simulink model "lyapunov_controller"  (R2016b)
settings: Solver=VariableStepAuto  StartTime=0.0  StopTime=200.0  RelTol=1e-3
libraries: simulink x2
settings Model: Creator=jocol  LastModifiedBy=jocol
settings DataIOCC: InspectSignalLogs=on

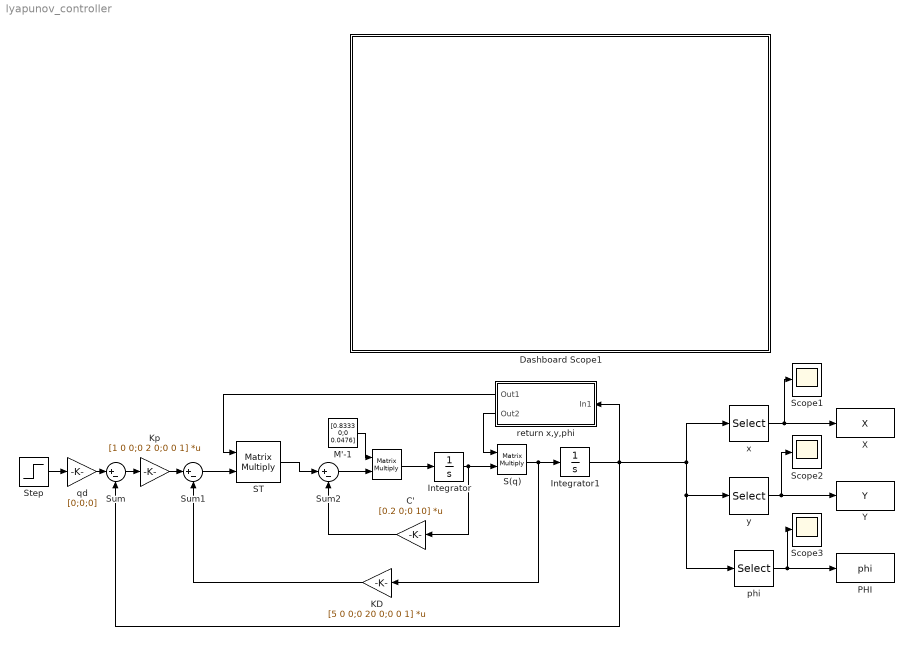
== system lyapunov_controller ==
  " " : Product  Multiplication=Matrix(*)
  C' : Gain  Gain=[0.2 0;0 10]  Multiplication=Matrix(K*u)
  Dashboard Scope1 : Subsystem  DialogController=hmiCreateDDGDialog  IsWebBlock=on  mask(MWDashboardBlock){webBlockId=055b4847-bd5b-4963-8916-93bab4c492f2, webBlockType=sdiscope, ShowInitialText=on, HMISrcModelName=untitled}
      mask prompts: webBlockId "WebBlock Id"; webBlockType "WebBlock Type"; HMISrcModelName "Source Model"
      mask help: SimulinkHMI:dialogs:HMIScopeDialogDesc
      mask Help: helpview([docroot '/mapfiles/simulink.map'], 'hmi_scope')
      mask Display:
      | if strcmp(get_param(bdroot(gcb),'BlockDiagramType'), 'library')
      |     image([(matlabroot) '/toolbox/simulink/hmi/icons/DashboardScope.png']);
      | end
  Integrator : Integrator
  Integrator1 : Integrator  InitialCondition=[7;7;-pi]
  KD : Gain  Gain=[5 0 0;0 20 0;0 0 1]  Multiplication=Matrix(K*u)
  Kp : Gain  Gain=[1 0 0;0 2 0;0 0 1]  Multiplication=Matrix(K*u)
  M'-1 : Constant  Value=[0.8333 0;0 0.0476]
  PHI : ToWorkspace  VariableName=phi  SaveFormat=Timeseries  SampleTime=-1
  S(q) : Product  Multiplication=Matrix(*)
  ST : Product  Multiplication=Matrix(*)
  Scope1 : Scope
  Scope2 : Scope
  Scope3 : Scope
  Step : Step  SampleTime=0
  Sum : Sum  Inputs=|+-
  Sum1 : Sum  Inputs=|+-
  Sum2 : Sum  Inputs=|+-
  X : ToWorkspace  VariableName=X  SaveFormat=Timeseries  SampleTime=-1
  Y : ToWorkspace  VariableName=Y  SaveFormat=Timeseries  SampleTime=-1
  phi : Selector  InputPortWidth=3  IndexOptions=Index vector (dialog)  Indices=3  OutputSizes=1
  qd : Gain  Gain=[0;0;0]
  return x,y,phi : Subsystem
  x : Selector  InputPortWidth=3  IndexOptions=Index vector (dialog)  Indices=1  OutputSizes=1
  y : Selector  InputPortWidth=3  IndexOptions=Index vector (dialog)  Indices=2  OutputSizes=1
  wires:
  Kp/1 -> Sum1/1
  Sum/1 -> Kp/1
  M'-1/1 -> " "/1
  Sum2/1 -> " "/2
  " "/1 -> Integrator/1
  Integrator/1 -> C'/1, S(q)/2
  C'/1 -> Sum2/2
  S(q)/1 -> KD/1, Integrator1/1
  KD/1 -> Sum1/2
  Sum1/1 -> ST/2
  ST/1 -> Sum2/1
  Step/1 -> qd/1
  qd/1 -> Sum/1
  x/1 -> Scope1/1, X/1
  y/1 -> Scope2/1, Y/1
  phi/1 -> Scope3/1, PHI/1
  return x,y,phi/1(Out1) -> ST/1
  return x,y,phi/2(Out2) -> S(q)/1
  Integrator1/1 -> phi/1, y/1, x/1, return x,y,phi/1(In1), Sum/2

== system lyapunov_controller/Dashboard Scope1 ==

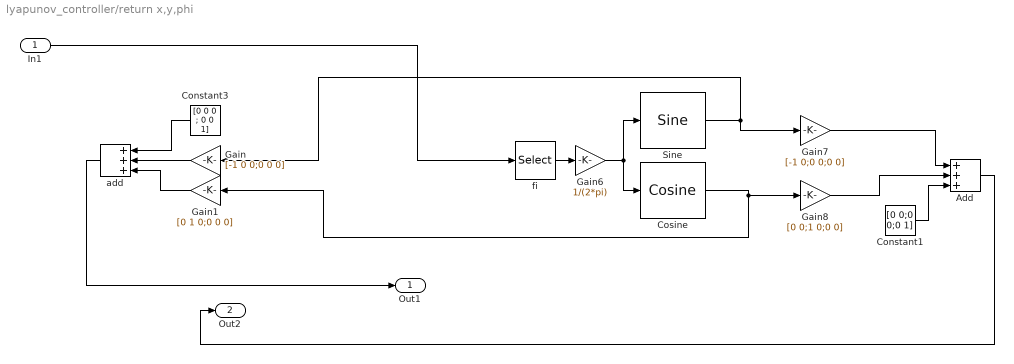
== system lyapunov_controller/return x,y,phi ==
  In1 : Inport
  Add : Sum  Inputs=+++
  Constant1 : Constant  Value=[0 0;0 0;0 1]
  Constant3 : Constant  Value=[0 0 0 ; 0 0 1]
  Cosine : simulink/Lookup Tables/Cosine  Formula=cos(2*pi*u)  NumDataPoints=(2^5)+1  OutputWordLength=16  InternalRulePriority=Speed
  Gain : Gain  Gain=[-1 0 0;0 0 0]
  Gain1 : Gain  Gain=[0 1 0;0 0 0]
  Gain6 : Gain  Gain=1/(2*pi)
  Gain7 : Gain  Gain=[-1 0;0 0;0 0]
  Gain8 : Gain  Gain=[0 0;1 0;0 0]
  Sine : simulink/Lookup Tables/Sine  Formula=sin(2*pi*u)  NumDataPoints=(2^5)+1  OutputWordLength=16  InternalRulePriority=Speed
  add : Sum  Inputs=+++
  fi : Selector  InputPortWidth=3  IndexOptions=Index vector (dialog)  Indices=3  OutputSizes=1
  Out1 : Outport
  Out2 : Outport  Port=2
  wires:
  In1/1 -> fi/1
  fi/1 -> Gain6/1
  Gain6/1 -> Cosine/1, Sine/1
  Gain7/1 -> Add/1
  Gain8/1 -> Add/2
  Constant1/1 -> Add/3
  Sine/1 -> Gain7/1, Gain/1
  Cosine/1 -> Gain1/1, Gain8/1
  Constant3/1 -> add/1
  Gain/1 -> add/2
  Gain1/1 -> add/3
  Add/1 -> Out2/1
  add/1 -> Out1/1
